simulink model "project"  (R2018b)
settings: Solver=VariableStepAuto  StartTime=0.0  StopTime=10.0  RelTol=1e-3
libraries: commutil2 x11
settings Model: Creator=Reza  LastModifiedBy=Rahmat

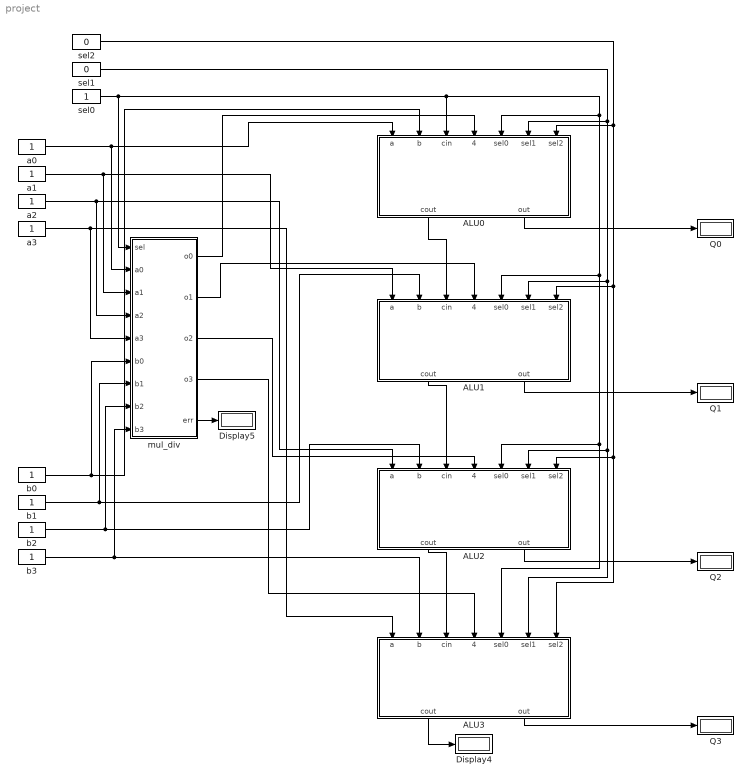
== system project ==
  ALU0 : Subsystem
  ALU1 : Subsystem
  ALU2 : Subsystem
  ALU3 : Subsystem
  Display4 : Display
  Display5 : Display
  Q{0..3} (4 alike) : Display
  a{0..3} (4 alike) : Constant
  b{0..3} (4 alike) : Constant
  mul_div : Subsystem
  sel0 : Constant
  sel1 : Constant  Value=0
  sel2 : Constant  Value=0
  wires:
  mul_div/1(o0) -> ALU0/4(mul_div)
  mul_div/2(o1) -> ALU1/4(mul_div)
  mul_div/3(o2) -> ALU2/4(mul_div)
  mul_div/4(o3) -> ALU3/4(mul_div)
  ALU0/1(cout) -> ALU1/3(cin)
  ALU1/1(cout) -> ALU2/3(cin)
  ALU2/1(cout) -> ALU3/3(cin)
  ALU0/2(out) -> Q0/1
  ALU1/2(out) -> Q1/1
  ALU2/2(out) -> Q2/1
  ALU3/2(out) -> Q3/1
  ALU3/1(cout) -> Display4/1
  mul_div/5(err) -> Display5/1
  sel0/1 -> mul_div/1(sel), ALU0/3(cin), ALU0/5(sel0), ALU1/5(sel0), ALU3/5(sel0), ALU2/5(sel0)
  sel1/1 -> ALU0/6(sel1), ALU1/6(sel1), ALU2/6(sel1), ALU3/6(sel1)
  sel2/1 -> ALU0/7(sel2), ALU1/7(sel2), ALU2/7(sel2), ALU3/7(sel2)
  a0/1 -> ALU0/1(a), mul_div/2(a0)
  a1/1 -> mul_div/3(a1), ALU1/1(a)
  a2/1 -> mul_div/4(a2), ALU2/1(a)
  a3/1 -> mul_div/5(a3), ALU3/1(a)
  b0/1 -> ALU0/2(b), mul_div/6(b0)
  b1/1 -> ALU1/2(b), mul_div/7(b1)
  b2/1 -> ALU2/2(b), mul_div/8(b2)
  b3/1 -> ALU3/2(b), mul_div/9(b3)

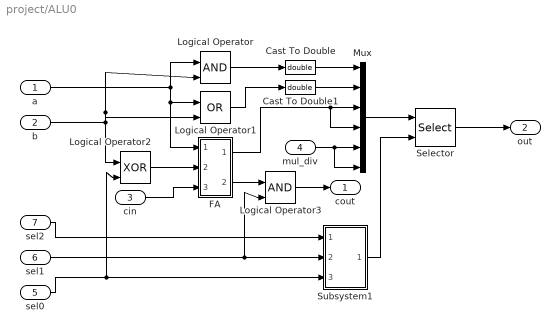
== system project/ALU0 ==
  a : Inport
  b : Inport  Port=2
  cin : Inport  Port=3
  mul_div : Inport  Port=4
  sel0 : Inport  Port=5
  sel1 : Inport  Port=6
  sel2 : Inport  Port=7
  Cast To Double : DataTypeConversion  OutDataTypeStr=double
  Cast To Double1 : DataTypeConversion  OutDataTypeStr=double
  FA : Subsystem
  Logical Operator : Logic  IconShape=distinctive  AllPortsSameDT=off  OutDataTypeStr=boolean
  Logical Operator1 : Logic  Operator=OR  IconShape=distinctive  AllPortsSameDT=off  OutDataTypeStr=boolean
  Logical Operator2 : Logic  Operator=XOR  IconShape=distinctive  AllPortsSameDT=off  OutDataTypeStr=boolean
  Logical Operator3 : Logic  IconShape=distinctive  AllPortsSameDT=off  OutDataTypeStr=boolean
  Mux : Mux  Inputs=6
  Selector : Selector  InputPortWidth=6  IndexOptions=Starting index (port)  Indices=[1 3]  OutputSizes=1
  Subsystem1 : Subsystem
  cout : Outport
  out : Outport  Port=2
  wires:
  b/1 -> Logical Operator/2, Logical Operator1/2, Logical Operator2/1
  Mux/1 -> Selector/1
  sel1/1 -> Logical Operator3/2, Subsystem1/2(sel1)
  FA/1(Out2) -> Mux/3, Mux/4
  sel2/1 -> Subsystem1/1(sel2)
  Subsystem1/1(Out1) -> Selector/2
  a/1 -> FA/1(In2), Logical Operator1/1, Logical Operator/1
  cin/1 -> FA/3(In4)
  Logical Operator2/1 -> FA/2(In3)
  Selector/1 -> out/1
  sel0/1 -> Logical Operator2/2, Subsystem1/3(sel0)
  Cast To Double1/1 -> Mux/2
  Cast To Double/1 -> Mux/1
  Logical Operator/1 -> Cast To Double/1
  Logical Operator1/1 -> Cast To Double1/1
  mul_div/1 -> Mux/5, Mux/6
  FA/2(Out1) -> Logical Operator3/1
  Logical Operator3/1 -> cout/1

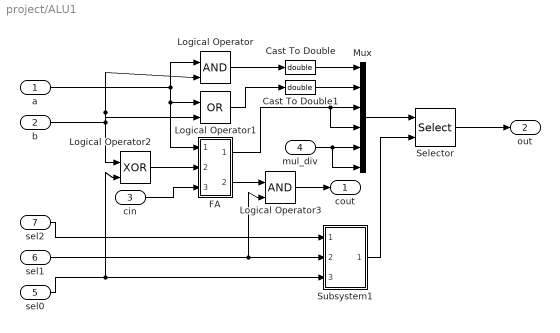
== system project/ALU1 ==
  a : Inport
  b : Inport  Port=2
  cin : Inport  Port=3
  mul_div : Inport  Port=4
  sel0 : Inport  Port=5
  sel1 : Inport  Port=6
  sel2 : Inport  Port=7
  Cast To Double : DataTypeConversion  OutDataTypeStr=double
  Cast To Double1 : DataTypeConversion  OutDataTypeStr=double
  FA : Subsystem
  Logical Operator : Logic  IconShape=distinctive  AllPortsSameDT=off  OutDataTypeStr=boolean
  Logical Operator1 : Logic  Operator=OR  IconShape=distinctive  AllPortsSameDT=off  OutDataTypeStr=boolean
  Logical Operator2 : Logic  Operator=XOR  IconShape=distinctive  AllPortsSameDT=off  OutDataTypeStr=boolean
  Logical Operator3 : Logic  IconShape=distinctive  AllPortsSameDT=off  OutDataTypeStr=boolean
  Mux : Mux  Inputs=6
  Selector : Selector  InputPortWidth=6  IndexOptions=Starting index (port)  Indices=[1 3]  OutputSizes=1
  Subsystem1 : Subsystem
  cout : Outport
  out : Outport  Port=2
  wires:
  b/1 -> Logical Operator/2, Logical Operator1/2, Logical Operator2/1
  Mux/1 -> Selector/1
  sel1/1 -> Logical Operator3/2, Subsystem1/2(sel1)
  FA/1(Out2) -> Mux/4, Mux/3
  sel2/1 -> Subsystem1/1(sel2)
  Subsystem1/1(Out1) -> Selector/2
  a/1 -> FA/1(In2), Logical Operator1/1, Logical Operator/1
  cin/1 -> FA/3(In4)
  sel0/1 -> Logical Operator2/2, Subsystem1/3(sel0)
  Logical Operator2/1 -> FA/2(In3)
  Selector/1 -> out/1
  Cast To Double/1 -> Mux/1
  Logical Operator/1 -> Cast To Double/1
  Cast To Double1/1 -> Mux/2
  Logical Operator1/1 -> Cast To Double1/1
  mul_div/1 -> Mux/6, Mux/5
  FA/2(Out1) -> Logical Operator3/1
  Logical Operator3/1 -> cout/1

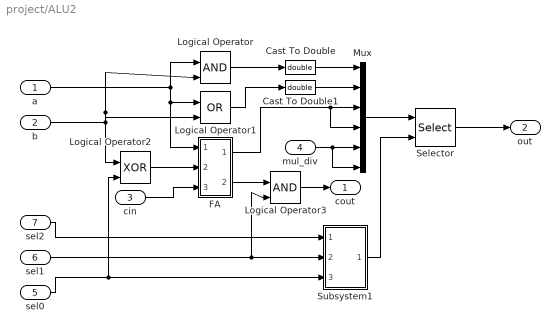
== system project/ALU2 ==
  a : Inport
  b : Inport  Port=2
  cin : Inport  Port=3
  mul_div : Inport  Port=4
  sel0 : Inport  Port=5
  sel1 : Inport  Port=6
  sel2 : Inport  Port=7
  Cast To Double : DataTypeConversion  OutDataTypeStr=double
  Cast To Double1 : DataTypeConversion  OutDataTypeStr=double
  FA : Subsystem
  Logical Operator : Logic  IconShape=distinctive  AllPortsSameDT=off  OutDataTypeStr=boolean
  Logical Operator1 : Logic  Operator=OR  IconShape=distinctive  AllPortsSameDT=off  OutDataTypeStr=boolean
  Logical Operator2 : Logic  Operator=XOR  IconShape=distinctive  AllPortsSameDT=off  OutDataTypeStr=boolean
  Logical Operator3 : Logic  IconShape=distinctive  AllPortsSameDT=off  OutDataTypeStr=boolean
  Mux : Mux  Inputs=6
  Selector : Selector  InputPortWidth=6  IndexOptions=Starting index (port)  Indices=[1 3]  OutputSizes=1
  Subsystem1 : Subsystem
  cout : Outport
  out : Outport  Port=2
  wires:
  b/1 -> Logical Operator/2, Logical Operator1/2, Logical Operator2/1
  Mux/1 -> Selector/1
  sel1/1 -> Logical Operator3/2, Subsystem1/2(sel1)
  FA/1(Out2) -> Mux/4, Mux/3
  sel2/1 -> Subsystem1/1(sel2)
  Subsystem1/1(Out1) -> Selector/2
  a/1 -> FA/1(In2), Logical Operator1/1, Logical Operator/1
  cin/1 -> FA/3(In4)
  sel0/1 -> Logical Operator2/2, Subsystem1/3(sel0)
  Logical Operator2/1 -> FA/2(In3)
  Selector/1 -> out/1
  Logical Operator/1 -> Cast To Double/1
  Cast To Double1/1 -> Mux/2
  Logical Operator1/1 -> Cast To Double1/1
  Cast To Double/1 -> Mux/1
  mul_div/1 -> Mux/5, Mux/6
  Logical Operator3/1 -> cout/1
  FA/2(Out1) -> Logical Operator3/1

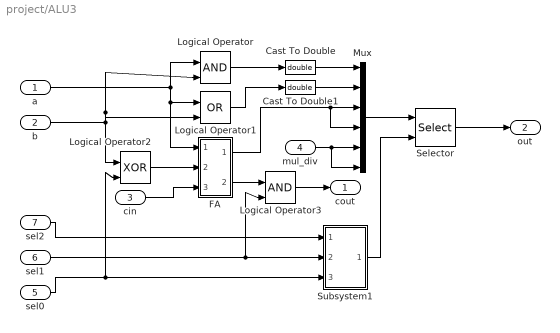
== system project/ALU3 ==
  a : Inport
  b : Inport  Port=2
  cin : Inport  Port=3
  mul_div : Inport  Port=4
  sel0 : Inport  Port=5
  sel1 : Inport  Port=6
  sel2 : Inport  Port=7
  Cast To Double : DataTypeConversion  OutDataTypeStr=double
  Cast To Double1 : DataTypeConversion  OutDataTypeStr=double
  FA : Subsystem
  Logical Operator : Logic  IconShape=distinctive  AllPortsSameDT=off  OutDataTypeStr=boolean
  Logical Operator1 : Logic  Operator=OR  IconShape=distinctive  AllPortsSameDT=off  OutDataTypeStr=boolean
  Logical Operator2 : Logic  Operator=XOR  IconShape=distinctive  AllPortsSameDT=off  OutDataTypeStr=boolean
  Logical Operator3 : Logic  IconShape=distinctive  AllPortsSameDT=off  OutDataTypeStr=boolean
  Mux : Mux  Inputs=6
  Selector : Selector  InputPortWidth=6  IndexOptions=Starting index (port)  Indices=[1 3]  OutputSizes=1
  Subsystem1 : Subsystem
  cout : Outport
  out : Outport  Port=2
  wires:
  b/1 -> Logical Operator/2, Logical Operator1/2, Logical Operator2/1
  Mux/1 -> Selector/1
  sel1/1 -> Logical Operator3/2, Subsystem1/2(sel1)
  FA/1(Out2) -> Mux/4, Mux/3
  sel2/1 -> Subsystem1/1(sel2)
  Subsystem1/1(Out1) -> Selector/2
  a/1 -> FA/1(In2), Logical Operator1/1, Logical Operator/1
  cin/1 -> FA/3(In4)
  sel0/1 -> Logical Operator2/2, Subsystem1/3(sel0)
  Logical Operator2/1 -> FA/2(In3)
  Selector/1 -> out/1
  Logical Operator/1 -> Cast To Double/1
  Cast To Double1/1 -> Mux/2
  Logical Operator1/1 -> Cast To Double1/1
  Cast To Double/1 -> Mux/1
  mul_div/1 -> Mux/6, Mux/5
  Logical Operator3/1 -> cout/1
  FA/2(Out1) -> Logical Operator3/1

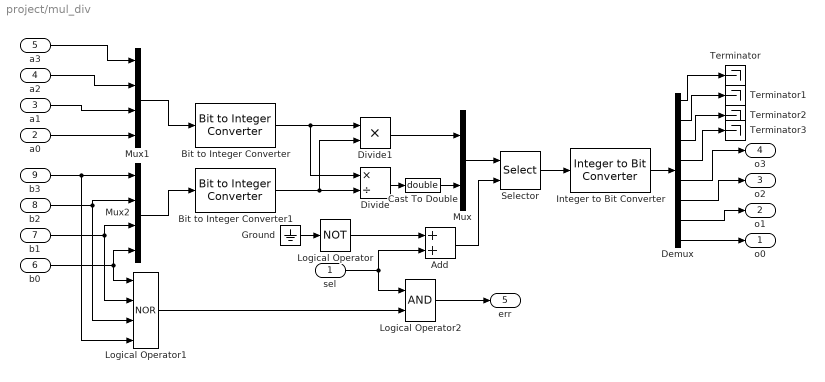
== system project/mul_div ==
  sel : Inport
  a0 : Inport  Port=2
  a1 : Inport  Port=3
  a2 : Inport  Port=4
  a3 : Inport  Port=5
  b0 : Inport  Port=6
  b1 : Inport  Port=7
  b2 : Inport  Port=8
  b3 : Inport  Port=9
  Add : Sum
  Bit to Integer Converter : commutil2/Bit to Integer Converter  nbits=4  bitOrder=MSB first  signedOutputValues=Unsigned  outDtype=Inherit via internal rule  outDtypeSigned=Inherit via internal rule
  Bit to Integer Converter1 : commutil2/Bit to Integer Converter  nbits=4  bitOrder=MSB first  signedOutputValues=Unsigned  outDtype=Inherit via internal rule  outDtypeSigned=Inherit via internal rule
  Cast To Double : DataTypeConversion  OutDataTypeStr=double
  Demux : Demux  Outputs=8
  Divide : Product  Inputs=*/  OutDataTypeStr=int32
  Divide1 : Product  Inputs=**
  Ground : Ground
  Integer to Bit Converter : commutil2/Integer to Bit Converter  nbits=8  signedInputValues=Unsigned  bitOrder=MSB first  outDtype=Inherit via internal rule
  Logical Operator : Logic  Operator=NOT  IconShape=distinctive  AllPortsSameDT=off  OutDataTypeStr=boolean
  Logical Operator1 : Logic  Operator=NOR  Inputs=4  IconShape=distinctive  AllPortsSameDT=off  OutDataTypeStr=boolean
  Logical Operator2 : Logic  IconShape=distinctive  AllPortsSameDT=off  OutDataTypeStr=boolean
  Mux : Mux  Inputs=2
  Mux1 : Mux
  Mux2 : Mux
  Selector : Selector  InputPortWidth=2  IndexOptions=Starting index (port)  Indices=[1 3]  OutputSizes=1
  Terminator{,1..3} (4 alike) : Terminator
  o0 : Outport
  o1 : Outport  Port=2
  o2 : Outport  Port=3
  o3 : Outport  Port=4
  err : Outport  Port=5
  wires:
  Logical Operator/1 -> Add/1
  a0/1 -> Mux1/4
  Divide1/1 -> Mux/1
  a1/1 -> Mux1/3
  Mux/1 -> Selector/1
  Bit to Integer Converter/1 -> Divide/1, Divide1/1
  a3/1 -> Mux1/1
  b3/1 -> Logical Operator1/4, Mux2/1
  Selector/1 -> Integer to Bit Converter/1
  b2/1 -> Mux2/2, Logical Operator1/3
  Integer to Bit Converter/1 -> Demux/1
  Bit to Integer Converter1/1 -> Divide/2, Divide1/2
  Mux2/1 -> Bit to Integer Converter1/1
  Mux1/1 -> Bit to Integer Converter/1
  Demux/4 -> Terminator3/1
  Add/1 -> Selector/2
  b0/1 -> Mux2/4, Logical Operator1/1
  Ground/1 -> Logical Operator/1
  b1/1 -> Mux2/3, Logical Operator1/2
  Demux/5 -> o3/1
  Demux/8 -> o0/1
  Demux/6 -> o2/1
  Demux/7 -> o1/1
  Demux/1 -> Terminator/1
  sel/1 -> Logical Operator2/1, Add/2
  a2/1 -> Mux1/2
  Demux/3 -> Terminator2/1
  Demux/2 -> Terminator1/1
  Divide/1 -> Cast To Double/1
  Cast To Double/1 -> Mux/2
  Logical Operator1/1 -> Logical Operator2/2
  Logical Operator2/1 -> err/1

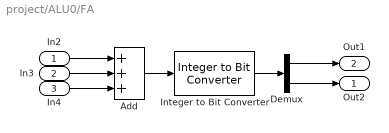
== system project/ALU0/FA ==
  In2 : Inport
  In3 : Inport  Port=2
  In4 : Inport  Port=3
  Add : Sum  Inputs=+++
  Demux : Demux  Outputs=2
  Integer to Bit Converter : commutil2/Integer to Bit Converter  nbits=2  signedInputValues=Unsigned  bitOrder=MSB first  outDtype=Inherit via internal rule
  Out2 : Outport
  Out1 : Outport  Port=2
  wires:
  Add/1 -> Integer to Bit Converter/1
  Integer to Bit Converter/1 -> Demux/1
  In4/1 -> Add/3
  In2/1 -> Add/1
  Demux/1 -> Out1/1
  In3/1 -> Add/2
  Demux/2 -> Out2/1

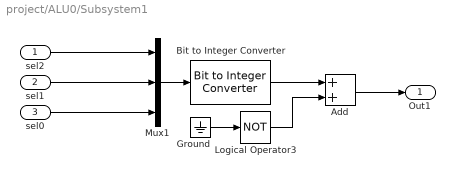
== system project/ALU0/Subsystem1 ==
  sel2 : Inport
  sel1 : Inport  Port=2
  sel0 : Inport  Port=3
  Add : Sum
  Bit to Integer Converter : commutil2/Bit to Integer Converter  nbits=3  bitOrder=MSB first  signedOutputValues=Unsigned  outDtype=Inherit via internal rule  outDtypeSigned=Inherit via internal rule
  Ground : Ground
  Logical Operator3 : Logic  Operator=NOT  IconShape=distinctive  AllPortsSameDT=off  OutDataTypeStr=boolean
  Mux1 : Mux  Inputs=3
  Out1 : Outport
  wires:
  sel0/1 -> Mux1/3
  Ground/1 -> Logical Operator3/1
  Bit to Integer Converter/1 -> Add/1
  sel1/1 -> Mux1/2
  Mux1/1 -> Bit to Integer Converter/1
  Add/1 -> Out1/1
  Logical Operator3/1 -> Add/2
  sel2/1 -> Mux1/1

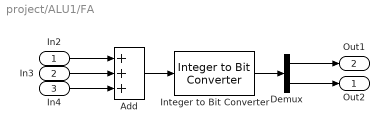
== system project/ALU1/FA ==
  In2 : Inport
  In3 : Inport  Port=2
  In4 : Inport  Port=3
  Add : Sum  Inputs=+++
  Demux : Demux  Outputs=2
  Integer to Bit Converter : commutil2/Integer to Bit Converter  nbits=2  signedInputValues=Unsigned  bitOrder=MSB first  outDtype=Inherit via internal rule
  Out2 : Outport
  Out1 : Outport  Port=2
  wires:
  Add/1 -> Integer to Bit Converter/1
  Integer to Bit Converter/1 -> Demux/1
  In4/1 -> Add/3
  In2/1 -> Add/1
  Demux/1 -> Out1/1
  In3/1 -> Add/2
  Demux/2 -> Out2/1

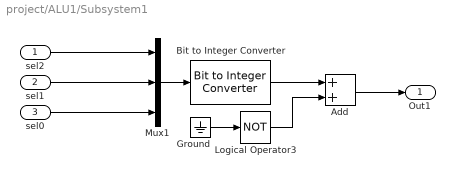
== system project/ALU1/Subsystem1 ==
  sel2 : Inport
  sel1 : Inport  Port=2
  sel0 : Inport  Port=3
  Add : Sum
  Bit to Integer Converter : commutil2/Bit to Integer Converter  nbits=3  bitOrder=MSB first  signedOutputValues=Unsigned  outDtype=Inherit via internal rule  outDtypeSigned=Inherit via internal rule
  Ground : Ground
  Logical Operator3 : Logic  Operator=NOT  IconShape=distinctive  AllPortsSameDT=off  OutDataTypeStr=boolean
  Mux1 : Mux  Inputs=3
  Out1 : Outport
  wires:
  sel0/1 -> Mux1/3
  Ground/1 -> Logical Operator3/1
  Bit to Integer Converter/1 -> Add/1
  sel1/1 -> Mux1/2
  Mux1/1 -> Bit to Integer Converter/1
  Add/1 -> Out1/1
  Logical Operator3/1 -> Add/2
  sel2/1 -> Mux1/1

== system project/ALU2/FA ==
  In2 : Inport
  In3 : Inport  Port=2
  In4 : Inport  Port=3
  Add : Sum  Inputs=+++
  Demux : Demux  Outputs=2
  Integer to Bit Converter : commutil2/Integer to Bit Converter  nbits=2  signedInputValues=Unsigned  bitOrder=MSB first  outDtype=Inherit via internal rule
  Out2 : Outport
  Out1 : Outport  Port=2
  wires:
  Add/1 -> Integer to Bit Converter/1
  Integer to Bit Converter/1 -> Demux/1
  In4/1 -> Add/3
  In2/1 -> Add/1
  Demux/1 -> Out1/1
  In3/1 -> Add/2
  Demux/2 -> Out2/1

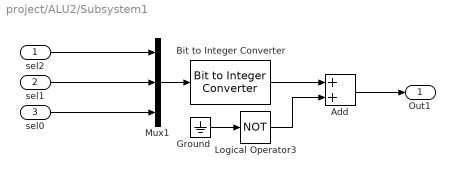
== system project/ALU2/Subsystem1 ==
  sel2 : Inport
  sel1 : Inport  Port=2
  sel0 : Inport  Port=3
  Add : Sum
  Bit to Integer Converter : commutil2/Bit to Integer Converter  nbits=3  bitOrder=MSB first  signedOutputValues=Unsigned  outDtype=Inherit via internal rule  outDtypeSigned=Inherit via internal rule
  Ground : Ground
  Logical Operator3 : Logic  Operator=NOT  IconShape=distinctive  AllPortsSameDT=off  OutDataTypeStr=boolean
  Mux1 : Mux  Inputs=3
  Out1 : Outport
  wires:
  sel0/1 -> Mux1/3
  Ground/1 -> Logical Operator3/1
  Bit to Integer Converter/1 -> Add/1
  sel1/1 -> Mux1/2
  Mux1/1 -> Bit to Integer Converter/1
  Add/1 -> Out1/1
  Logical Operator3/1 -> Add/2
  sel2/1 -> Mux1/1

== system project/ALU3/FA ==
  In2 : Inport
  In3 : Inport  Port=2
  In4 : Inport  Port=3
  Add : Sum  Inputs=+++
  Demux : Demux  Outputs=2
  Integer to Bit Converter : commutil2/Integer to Bit Converter  nbits=2  signedInputValues=Unsigned  bitOrder=MSB first  outDtype=Inherit via internal rule
  Out2 : Outport
  Out1 : Outport  Port=2
  wires:
  Add/1 -> Integer to Bit Converter/1
  Integer to Bit Converter/1 -> Demux/1
  In4/1 -> Add/3
  In2/1 -> Add/1
  Demux/1 -> Out1/1
  In3/1 -> Add/2
  Demux/2 -> Out2/1

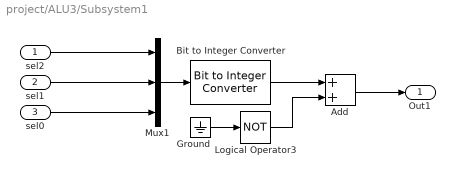
== system project/ALU3/Subsystem1 ==
  sel2 : Inport
  sel1 : Inport  Port=2
  sel0 : Inport  Port=3
  Add : Sum
  Bit to Integer Converter : commutil2/Bit to Integer Converter  nbits=3  bitOrder=MSB first  signedOutputValues=Unsigned  outDtype=Inherit via internal rule  outDtypeSigned=Inherit via internal rule
  Ground : Ground
  Logical Operator3 : Logic  Operator=NOT  IconShape=distinctive  AllPortsSameDT=off  OutDataTypeStr=boolean
  Mux1 : Mux  Inputs=3
  Out1 : Outport
  wires:
  sel0/1 -> Mux1/3
  Ground/1 -> Logical Operator3/1
  Bit to Integer Converter/1 -> Add/1
  sel1/1 -> Mux1/2
  Mux1/1 -> Bit to Integer Converter/1
  Add/1 -> Out1/1
  Logical Operator3/1 -> Add/2
  sel2/1 -> Mux1/1
